simulink model "SIMULATION_OF_MPC_AND_ISP"  (R2022a)
settings: Solver=FixedStepDiscrete  StartTime=0.0  StopTime=6  FixedStep=1/500  RelTol=1e-3
libraries: eeStairGenerator x1
settings Model: Creator=minhk  LastModifiedBy=minhk

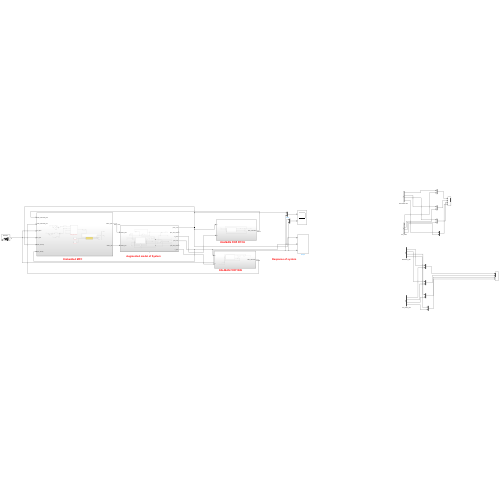
[thumbnail: Simulink's stored preview of the top-level diagram]
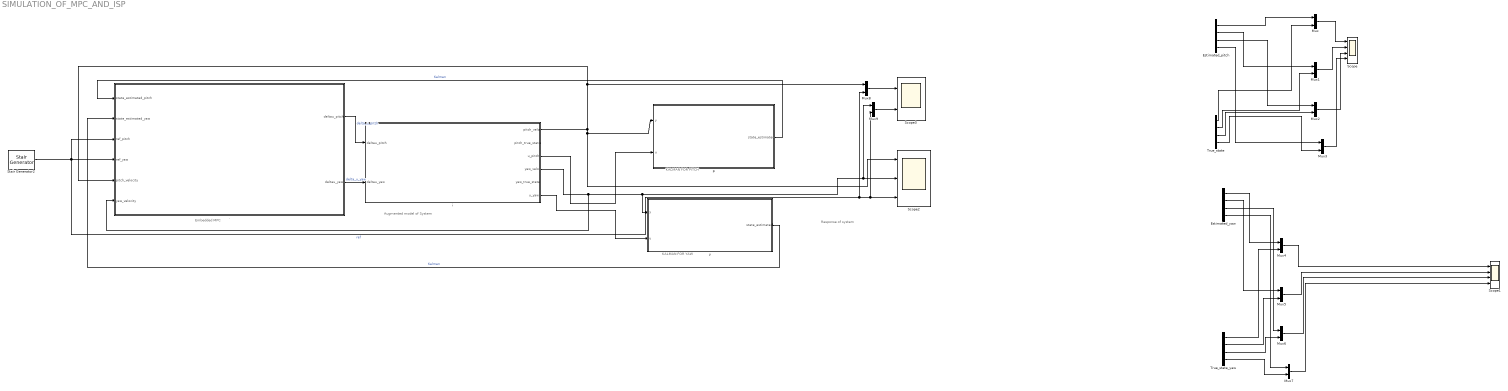
== system SIMULATION_OF_MPC_AND_ISP ==
  note: KALMAN FOR PITCH
  note: Embedded MPC
  note: Augmented model of System
  note: KALMAN FOR YAW
  note: Response of system
  . : Subsystem
  Estimated_pitch : Demux
  Estimated_yaw : Demux
  Mux{,1..9} (10 alike) : Mux  Inputs=2
  Scope : Scope  NumInputPorts=4
  Scope1 : Scope  NumInputPorts=4
  Scope2 : Scope  NumInputPorts=3
  Scope3 : Scope  NumInputPorts=2
  Stair Generator2 : eeStairGenerator/Stair Generator  LabelModeActiveChoice=Discrete  TimeInput=[1 2 3 4 5 6]  AmplitudeInput=[0 1 -1 1 -2 3]  SampleTime=1/500  RepeatPattern=off  OutDataTypeStr=double
      settings: SourceProductBaseCode=PS
  True_state : Demux
  True_state_yaw : Demux
  i : Subsystem
  p : Subsystem
  y : Subsystem
  wires:
  ./1(deltau_pitch) -> i/1(deltau_pitch)  "delta_u_pitch"
  ./2(deltau_yaw) -> i/2(deltau_yaw)  "delta_u_yaw"
  i/1(pitch_velo) -> p/1(y), Scope2/1, Mux8/1, ./5(pitch_velocity)
  i/3(u_pitch) -> p/2(u)
  Stair Generator2/1 -> ./3(ref_pitch), Mux8/2, Mux9/2, Scope2/3, ./4(ref_yaw)  "ref"
  Estimated_pitch/2 -> Mux1/1
  Estimated_pitch/3 -> Mux2/1
  Estimated_pitch/4 -> Mux3/1
  True_state/4 -> Mux3/2
  True_state/2 -> Mux1/2
  True_state/3 -> Mux2/2
  Estimated_pitch/1 -> Mux/1
  True_state/1 -> Mux/2
  Mux/1 -> Scope/1
  Mux1/1 -> Scope/2
  Mux2/1 -> Scope/3
  Mux3/1 -> Scope/4
  True_state_yaw/2 -> Mux5/2
  Mux7/1 -> Scope1/4
  True_state_yaw/3 -> Mux6/2
  True_state_yaw/4 -> Mux7/2
  Mux5/1 -> Scope1/2
  Mux6/1 -> Scope1/3
  Estimated_yaw/3 -> Mux6/1
  Estimated_yaw/2 -> Mux5/1
  Estimated_yaw/1 -> Mux4/1
  i/6(u_yaw) -> y/2(u)
  i/4(yaw_velo) -> Scope2/2, Mux9/1, y/1(y), ./6(yaw_velocity)
  Estimated_yaw/4 -> Mux7/1
  Mux4/1 -> Scope1/1
  True_state_yaw/1 -> Mux4/2
  p/1(state_estimated) -> ./1(state_estimated_pitch)  "Kalman"
  y/1(state_estimated) -> ./2(state_estimated_yaw)  "Kalman"
  Mux8/1 -> Scope3/1
  Mux9/1 -> Scope3/2

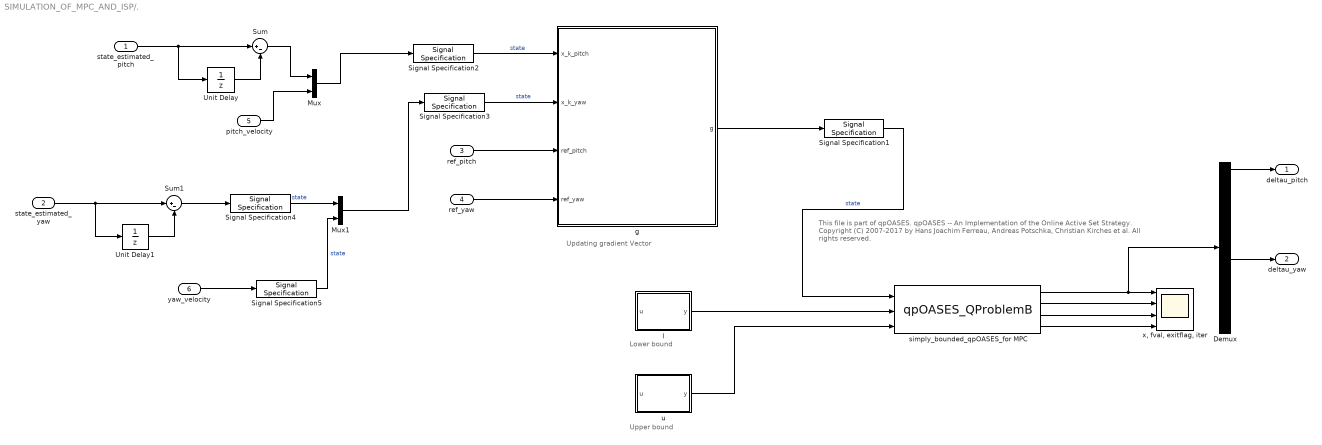
== system SIMULATION_OF_MPC_AND_ISP/. ==
  note: Lower bound
  note: This file is part of qpOASES.
      |
      | qpOASES -- An Implementation of the Online Active Set Strategy.
      | Copyright (C) 2007-2017 by Hans Joachim Ferreau, Andreas Potschka, Christian Kirches et al.
      | All rights reserved.
  note: Upper bound
  note: Updating gradient Vector
  state_estimated_pitch : Inport
  state_estimated_yaw : Inport  Port=2
  ref_pitch : Inport  Port=3
  ref_yaw : Inport  Port=4
  pitch_velocity : Inport  Port=5
  yaw_velocity : Inport  Port=6
  Demux : Demux  Outputs=8
  Mux : Mux  Inputs=2
  Mux1 : Mux  Inputs=2
  Signal Specification1 : SignalSpecification  Dimensions=8  SampleTime=1/500
  Signal Specification2 : SignalSpecification  Dimensions=5  SampleTime=1/500
  Signal Specification3 : SignalSpecification  Dimensions=5  SampleTime=1/500
  Signal Specification4 : SignalSpecification  Dimensions=4  SampleTime=1/500
  Signal Specification5 : SignalSpecification  Dimensions=1  SampleTime=1/500
  Sum : Sum  Inputs=|+-
  Sum1 : Sum  Inputs=|+-
  Unit Delay : UnitDelay  SampleTime=-1  HasFrameUpgradeWarning=on
  Unit Delay1 : UnitDelay  SampleTime=-1  HasFrameUpgradeWarning=on
  g : MATLAB Function  TreatAsAtomicUnit=on
  l : MATLAB Function  TreatAsAtomicUnit=on
  simply_bounded_qpOASES_for MPC : S-Function  FunctionName=qpOASES_QProblemB  Parameters=H_pitch_yaw  SFunctionDeploymentMode=off  EnableBusSupport=off
  u : MATLAB Function  TreatAsAtomicUnit=on
  "x, fval, exitflag, iter" : Scope  NumInputPorts=4
  deltau_pitch : Outport
  deltau_yaw : Outport  Port=2
  wires:
  simply_bounded_qpOASES_for MPC/4 -> "x, fval, exitflag, iter"/4
  simply_bounded_qpOASES_for MPC/3 -> "x, fval, exitflag, iter"/3
  u/1(y) -> simply_bounded_qpOASES_for MPC/3
  simply_bounded_qpOASES_for MPC/1 -> Demux/1, "x, fval, exitflag, iter"/1
  simply_bounded_qpOASES_for MPC/2 -> "x, fval, exitflag, iter"/2
  l/1(y) -> simply_bounded_qpOASES_for MPC/2
  g/1(g) -> Signal Specification1/1
  state_estimated_pitch/1 -> Sum/1, Unit Delay/1
  Demux/1 -> deltau_pitch/1
  Signal Specification1/1 -> simply_bounded_qpOASES_for MPC/1  "state"
  Demux/5 -> deltau_yaw/1
  ref_yaw/1 -> g/4(ref_yaw)
  ref_pitch/1 -> g/3(ref_pitch)
  Unit Delay/1 -> Sum/2
  Unit Delay1/1 -> Sum1/2
  state_estimated_yaw/1 -> Unit Delay1/1, Sum1/1
  Sum/1 -> Mux/1
  pitch_velocity/1 -> Mux/2
  Mux/1 -> Signal Specification2/1
  Sum1/1 -> Signal Specification4/1
  yaw_velocity/1 -> Signal Specification5/1
  Mux1/1 -> Signal Specification3/1
  Signal Specification2/1 -> g/1(x_k_pitch)  "state"
  Signal Specification3/1 -> g/2(x_k_yaw)  "state"
  Signal Specification4/1 -> Mux1/1  "state"
  Signal Specification5/1 -> Mux1/2  "state"

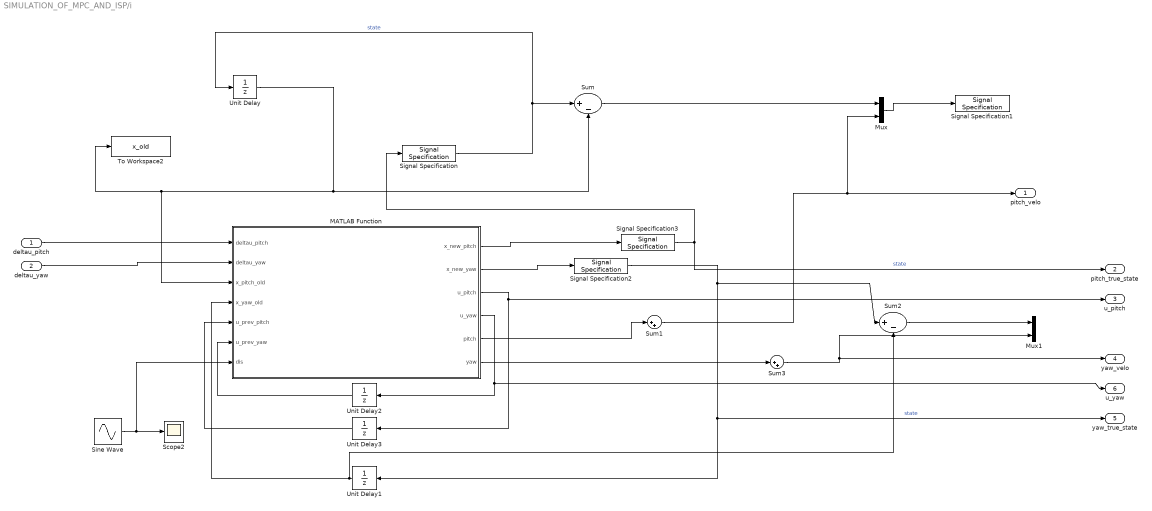
== system SIMULATION_OF_MPC_AND_ISP/i ==
  deltau_pitch : Inport
  deltau_yaw : Inport  Port=2
  MATLAB Function : MATLAB Function  TreatAsAtomicUnit=on
  Mux : Mux  Inputs=2
  Mux1 : Mux  Inputs=2
  Scope2 : Scope
  Signal Specification : SignalSpecification  Dimensions=4  SampleTime=1/500
  Signal Specification1 : SignalSpecification  Dimensions=5  SampleTime=1/500
  Signal Specification2 : SignalSpecification  Dimensions=4  SampleTime=1/500
  Signal Specification3 : SignalSpecification  Dimensions=4  SampleTime=1/500
  Sine Wave : Sin  Amplitude=2  Frequency=18  SampleTime=1/500
  Sum : Sum  Inputs=|+-
  Sum1 : Sum  Inputs=|++
  Sum2 : Sum  Inputs=|+-
  Sum3 : Sum  Inputs=|++
  To Workspace2 : ToWorkspace  VariableName=x_old  SampleTime=-1
      settings: Save2DSignal=2-D array (concatenate along first dimension)
  Unit Delay : UnitDelay  InitialCondition=[0;0;0;0]  SampleTime=1/500  HasFrameUpgradeWarning=on
  Unit Delay1 : UnitDelay  SampleTime=1/500  HasFrameUpgradeWarning=on
  Unit Delay2 : UnitDelay  SampleTime=1/500  HasFrameUpgradeWarning=on
  Unit Delay3 : UnitDelay  SampleTime=1/500  HasFrameUpgradeWarning=on
  pitch_velo : Outport
  pitch_true_state : Outport  Port=2
  u_pitch : Outport  Port=3
  yaw_velo : Outport  Port=4
  yaw_true_state : Outport  Port=5
  u_yaw : Outport  Port=6
  wires:
  Unit Delay/1 -> Sum/2, MATLAB Function/3(x_pitch_old), To Workspace2/1
  Signal Specification/1 -> Sum/1, Unit Delay/1  "state"
  Sum/1 -> Mux/1
  Mux/1 -> Signal Specification1/1
  MATLAB Function/2(x_new_yaw) -> Signal Specification2/1
  Sum2/1 -> Mux1/1
  MATLAB Function/1(x_new_pitch) -> Signal Specification3/1
  deltau_pitch/1 -> MATLAB Function/1(deltau_pitch)
  deltau_yaw/1 -> MATLAB Function/2(deltau_yaw)
  MATLAB Function/5(pitch) -> Sum1/1
  Unit Delay1/1 -> Sum2/2, MATLAB Function/4(x_yaw_old)
  MATLAB Function/6(yaw) -> Sum3/1
  MATLAB Function/4(u_yaw) -> Unit Delay2/1, u_yaw/1
  Unit Delay2/1 -> MATLAB Function/6(u_prev_yaw)
  MATLAB Function/3(u_pitch) -> u_pitch/1, Unit Delay3/1
  Unit Delay3/1 -> MATLAB Function/5(u_prev_pitch)
  Signal Specification2/1 -> yaw_true_state/1, Unit Delay1/1, Sum2/1  "state"
  Signal Specification3/1 -> pitch_true_state/1, Signal Specification/1  "state"
  Sine Wave/1 -> MATLAB Function/7(dis), Scope2/1
  Sum1/1 -> Mux/2, pitch_velo/1
  Sum3/1 -> yaw_velo/1, Mux1/2

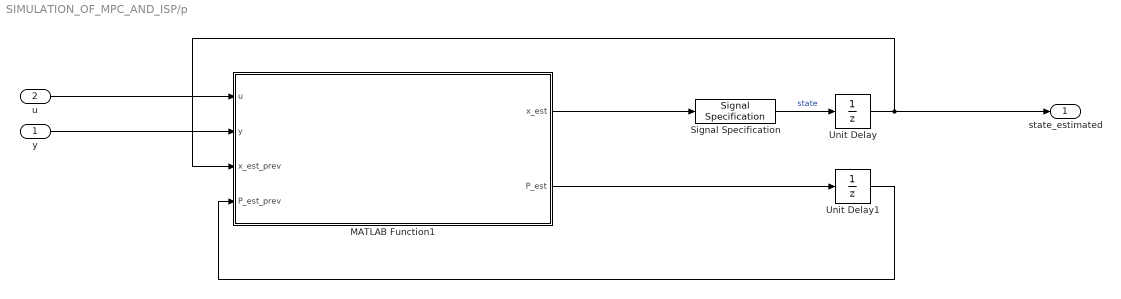
== system SIMULATION_OF_MPC_AND_ISP/p ==
  y : Inport
  u : Inport  Port=2
  MATLAB Function1 : MATLAB Function  TreatAsAtomicUnit=on
  Signal Specification : SignalSpecification  Dimensions=4  SampleTime=1/500
  Unit Delay : UnitDelay  SampleTime=-1  HasFrameUpgradeWarning=on
  Unit Delay1 : UnitDelay  SampleTime=-1  HasFrameUpgradeWarning=on
  state_estimated : Outport
  wires:
  MATLAB Function1/2(P_est) -> Unit Delay1/1
  Unit Delay1/1 -> MATLAB Function1/4(P_est_prev)
  y/1 -> MATLAB Function1/2(y)
  Unit Delay/1 -> state_estimated/1, MATLAB Function1/3(x_est_prev)
  MATLAB Function1/1(x_est) -> Signal Specification/1
  u/1 -> MATLAB Function1/1(u)
  Signal Specification/1 -> Unit Delay/1  "state"

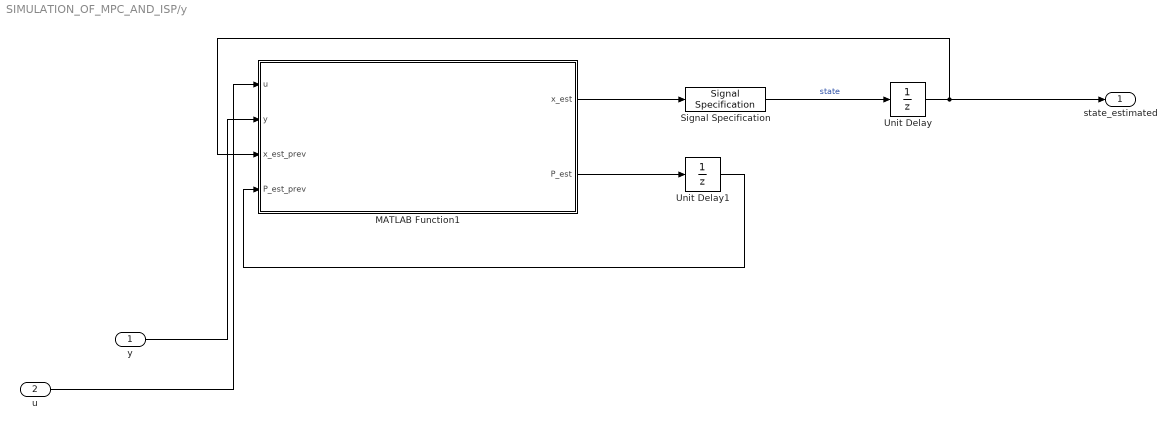
== system SIMULATION_OF_MPC_AND_ISP/y ==
  y : Inport
  u : Inport  Port=2
  MATLAB Function1 : MATLAB Function  TreatAsAtomicUnit=on
  Signal Specification : SignalSpecification  Dimensions=4  SampleTime=1/500
  Unit Delay : UnitDelay  SampleTime=-1  HasFrameUpgradeWarning=on
  Unit Delay1 : UnitDelay  SampleTime=-1  HasFrameUpgradeWarning=on
  state_estimated : Outport
  wires:
  MATLAB Function1/2(P_est) -> Unit Delay1/1
  Unit Delay1/1 -> MATLAB Function1/4(P_est_prev)
  y/1 -> MATLAB Function1/2(y)
  Unit Delay/1 -> state_estimated/1, MATLAB Function1/3(x_est_prev)
  MATLAB Function1/1(x_est) -> Signal Specification/1
  u/1 -> MATLAB Function1/1(u)
  Signal Specification/1 -> Unit Delay/1  "state"

== matlab function SIMULATION_OF_MPC_AND_ISP/y/MATLAB Function1 ==
  data: u input; x_est output; y input; P_est output; x_est_prev input; P_est_prev input
function [x_est, P_est] = kalmanFilter(u, y, x_est_prev, P_est_prev)
  A =  [0.8395358858304703     -0.04847432078257747   0.0                 0.0;
 0.0018635915154337373   0.9996816594546751   -0.5060644359497555  0.0;
 0.0                     0.01392345527731321   0.7448461065980053  0.3870783090569654;
 0.0                     0.0                  -0.4708561993095687  0.8385926646058729 ];
B = [-0.21792759566688183;
 -0.038489522945624556;
  0.011141404129424179;
 -0.034621154732298216];

H = [-0.15780307636762234  -0.04495569299225192  0.47795874838852487  0.8449536781870718];
Q = diag([1;23;23;1]);
R = 0.6;
    % Q - Process noise covariance matrix (NxN)
    % R - Measurement noise covariance matrix (MxM)
    % x_est_prev - Previous state estimate (Nx1 vector)
    % P_est_prev - Previous estimate covariance (NxN matrix)

    % Prediction Step:
    % Predicted state estimate (Nx1 vector)
    x_pred = A * x_est_prev + B * u;  % x_pred is Nx1
    
    % Predicted covariance estimate (NxN matrix)
    P_pred = A * P_est_prev * A' + Q; % P_pred is NxN

    % Update Step:
    % Kalman Gain (NxM matrix)
    K = P_pred * H' / (H * P_pred * H' + R);  % K is NxM
    
    % Measurement prediction (Mx1 vector)
    y_pred = H * x_pred;  % y_pred is Mx1
    
    % Measurement residual (Mx1 vector)
    y_residual = y - y_pred;  % y_residual is Mx1

    % Updated state estimate (Nx1 vector)
    x_est = x_pred + K * y_residual;  % x_est is Nx1
    
    % Updated covariance estimate (NxN matrix)
    P_est = (eye(size(K,1)) - K * H) * P_pred;  % P_est is NxN

== matlab function SIMULATION_OF_MPC_AND_ISP/./g ==
  data: x_k_pitch input; g output; x_k_yaw input; ref_pitch input; ref_yaw input
function g = fcn(x_k_pitch,x_k_yaw, ref_pitch, ref_yaw)

Phi_pitch = [-0.207898075873955	-0.0977583454820833	0.959319156000490	0.637943448418819	1;
-0.371399772311225	-0.179520448326943	1.47215082845275	1.24265429366304	1;
-0.504358581389858	-0.249073944262689	1.65960448278518	1.65246866768918	1;
-0.615226419955068	-0.308461239905408	1.69712008400333	1.86422966968891	1;
-0.708919237802465	-0.359174477397963	1.71381271201535	1.94919632847819	1;
-0.788568917299257	-0.402664279612529	1.76670271816044	1.98396399999896	1;
-0.856618765422683	-0.440389989599441	1.85900365181989	2.01717083871664	1;
-0.915268500689886	-0.473690907053775	1.97032520403141	2.06610579803703	1;
-0.966521340539038	-0.503666717080388	2.07956685177461	2.12804127657937	1;
-1.01209405046772	-0.531138410692773	2.17505711406798	2.19338688646969	1;];
Omega_pitch = [0.8	0	0	0	0	0	0	0	0	0;
0	0.8	0	0	0	0	0	0	0	0;
0	0	0.8	0	0	0	0	0	0	0;
0	0	0	0.8	0	0	0	0	0	0;
0	0	0	0	0.4	0	0	0	0	0;
0	0	0	0	0	0.4	0	0	0	0;
0	0	0	0	0	0	0.4	0	0	0;
0	0	0	0	0	0	0	0.4	0	0;
0	0	0	0	0	0	0	0	0.4	0;
0	0	0	0	0	0	0	0	0	1];

Ro_pitch = [-0.00437405731014054	0	0	0;
-0.00773738317456150	-0.00437405731014054	0	0;
0.0110305266523032	-0.00773738317456150	-0.00437405731014054	0;
0.0472674163101827	0.0110305266523032	-0.00773738317456150	-0.00437405731014054;
0.0879747037062141	0.0472674163101827	0.0110305266523032	-0.00773738317456150;
0.122765911075150	0.0879747037062141	0.0472674163101827	0.0110305266523032;
0.147410054261486	0.122765911075150	0.0879747037062141	0.0472674163101827;
0.162663543761580	0.147410054261486	0.122765911075150	0.0879747037062141;
0.171546692443707	0.162663543761580	0.147410054261486	0.122765911075150;
0.177103059860532	0.171546692443707	0.162663543761580	0.147410054261486];


Phi_yaw = [-0.132565124553096	-0.0306371475705194	-0.0190954872353023	0.893579420584644	1
-0.243915398953276	-0.0551044128851241	-0.438561725509457	1.63553711902003	1
-0.337443547197343	-0.0800066797655966	-1.08797288905037	2.09537112015816	1
-0.416010191636782	-0.109409353076817	-1.77559780424157	2.22961156538283	1
-0.482024503645489	-0.144568316353844	-2.33610084366897	2.07601992860402	1
-0.537511409500862	-0.184320227173043	-2.66347707506405	1.73026053993364	1
-0.584168739483869	-0.225928001590293	-2.72440200645982	1.31358901480221	1
-0.623416782237018	-0.266109133743053	-2.55253311882922	0.940588610852762	1
-0.656441803793855	-0.301981943627301	-2.22855345250895	0.694319926609283	1
-0.684234346785280	-0.331731551858121	-1.85312736946152	0.613206315888649	1];

% Ro_yaw = [-0.00437405731014054	0	0	0;
% -0.00773738317456150	-0.00437405731014054	0	0;
% 0.0110305266523032	-0.00773738317456150	-0.00437405731014054	0;
% 0.0472674163101827	0.0110305266523032	-0.00773738317456150	-0.00437405731014054;
% 0.0879747037062141	0.0472674163101827	0.0110305266523032	-0.00773738317456150;
% 0.122765911075150	0.0879747037062141	0.0472674163101827	0.0110305266523032;
% 0.147410054261486	0.122765911075150	0.0879747037062141	0.0472674163101827;
% 0.162663543761580	0.147410054261486	0.122765911075150	0.0879747037062141;
% 0.171546692443707	0.162663543761580	0.147410054261486	0.122765911075150;
% 0.177103059860532	0.171546692443707	0.162663543761580	0.147410054261486];
Ro_yaw = [0.0121918277374462	0	0	0;
0.0111111338689920	0.0121918277374462	0	0;
0.00595828965400074	0.0111111338689920	0.0121918277374462	0;
0.00414379417675620	0.00595828965400074	0.0111111338689920	0.0121918277374462;
0.0100886626730709	0.00414379417675620	0.00595828965400074	0.0111111338689920;
0.0249009836370022	0.0100886626730709	0.00414379417675620	0.00595828965400074;
0.0468463021036276	0.0249009836370022	0.0100886626730709	0.00414379417675620;
0.0723625452970900	0.0468463021036276	0.0249009836370022	0.0100886626730709;
0.0972908949316003	0.0723625452970900	0.0468463021036276	0.0249009836370022;
0.118004380430596	0.0972908949316003	0.0723625452970900	0.0468463021036276
    ];

x_k_pitch
g_pitch = 2*Ro_pitch'*Omega_pitch*(Phi_pitch*x_k_pitch - ref_pitch*ones(10,1));
g_yaw = 2*Ro_yaw'*Omega_pitch*(Phi_yaw*x_k_yaw - ref_yaw*ones(10,1));
g = [g_pitch;g_yaw];

== matlab function SIMULATION_OF_MPC_AND_ISP/./l ==
  data: u input; y output
function y = fcn(u)

y = -1000*ones(8,1);

== matlab function SIMULATION_OF_MPC_AND_ISP/./u ==
  data: u input; y output
function y = fcn(u)

y = 1000*ones(8,1);

== matlab function SIMULATION_OF_MPC_AND_ISP/i/MATLAB Function ==
  data: x_new_pitch output; x_new_yaw output; deltau_pitch input; u_pitch output; deltau_yaw input; x_pitch_old input; x_yaw_old input; u_yaw output; u_prev_pitch input; u_prev_yaw input; pitch output; yaw output; dis input
function [x_new_pitch,x_new_yaw,u_pitch, u_yaw,pitch,yaw] = fcn(deltau_pitch,deltau_yaw,x_pitch_old,x_yaw_old, u_prev_pitch,u_prev_yaw, dis)
A_pitch = [.36510488797294954  -0.2818303608478543     0.0                 0.0;
 0.8960574394292654    1.3762504151997674    -1.6750222787717166  0.0;
 0.0                  -0.006060682717179857   0.7071615442060207  0.41207960935436705;
 0.0                   0.0                   -0.5162046114370005  0.32823439556025524];
B_pitch = [ -1.0201806764501928;
  1.1740501247521735;
 -0.10944958687299033;
  0.0067613477039227205];
%F_m = [0.05  ;  0.05   ; 0.1  ;  0.05];
C_pitch = [-0.2722799907498721,-0.1210718371168788,1.2985249010575335,0.3133364932049975]; 

A_yaw =  [0.8395358858304703     -0.04847432078257747   0.0                 0.0;
 0.0018635915154337373   0.9996816594546751   -0.5060644359497555  0.0;
 0.0                     0.01392345527731321   0.7448461065980053  0.3870783090569654;
 0.0                     0.0                  -0.4708561993095687  0.8385926646058729 ];
B_yaw = [-0.21792759566688183;
 -0.038489522945624556;
  0.011141404129424179;
 -0.034621154732298216];
C_yaw = [-0.15780307636762234  -0.04495569299225192  0.47795874838852487  0.8449536781870718];
F_m_pitch = [0.05  ;  0.05   ; 0.1  ;  0.05];
F_m_yaw = [0.05  ;  0.05   ; 0.05  ;  0.1];

%D = [0];
u_pitch = u_prev_pitch + deltau_pitch; 
x_new_pitch = A_pitch*x_pitch_old + B_pitch*u_pitch + F_m_pitch*dis ;


u_yaw = u_prev_yaw + deltau_yaw; 
x_new_yaw = A_yaw*x_yaw_old + B_yaw*u_yaw + F_m_yaw*dis ;
%x_new_noise = A_m*x_old_noise + B_m*u + F_m*dis; 
%state_noise = A_m*x_old + B_m*u + F_m*d;

pitch = C_pitch*x_new_pitch;
yaw = C_yaw*x_new_yaw;
%y_noise = C_m*x_old_noise ;

== matlab function SIMULATION_OF_MPC_AND_ISP/p/MATLAB Function1 ==
  data: u input; x_est output; y input; P_est output; x_est_prev input; P_est_prev input
function [x_est, P_est] = kalmanFilter(u, y, x_est_prev, P_est_prev)
   A = [.36510488797294954  -0.2818303608478543     0.0                 0.0;
 0.8960574394292654    1.3762504151997674    -1.6750222787717166  0.0;
 0.0                  -0.006060682717179857   0.7071615442060207  0.41207960935436705;
 0.0                   0.0                   -0.5162046114370005  0.32823439556025524];
B = [ -1.0201806764501928;
  1.1740501247521735;
 -0.10944958687299033;
  0.0067613477039227205];
H = [-0.2722799907498721,-0.1210718371168788,1.2985249010575335,0.3133364932049975]; 
Q = diag([1;5;2.5;1]);
R = 0.06;
    % Q - Process noise covariance matrix (NxN)
    % R - Measurement noise covariance matrix (MxM)
    % x_est_prev - Previous state estimate (Nx1 vector)
    % P_est_prev - Previous estimate covariance (NxN matrix)

    % Prediction Step:
    % Predicted state estimate (Nx1 vector)
    x_pred = A * x_est_prev + B * u;  % x_pred is Nx1
    
    % Predicted covariance estimate (NxN matrix)
    P_pred = A * P_est_prev * A' + Q; % P_pred is NxN

    % Update Step:
    % Kalman Gain (NxM matrix)
    K = P_pred * H' / (H * P_pred * H' + R);  % K is NxM
    
    % Measurement prediction (Mx1 vector)
    y_pred = H * x_pred;  % y_pred is Mx1
    
    % Measurement residual (Mx1 vector)
    y_residual = y - y_pred;  % y_residual is Mx1

    % Updated state estimate (Nx1 vector)
    x_est = x_pred + K * y_residual;  % x_est is Nx1
    
    % Updated covariance estimate (NxN matrix)
    P_est = (eye(size(K,1)) - K * H) * P_pred;  % P_est is NxN
